simulink model "CARTESIAN_SPACE"  (R2021a)
settings: Solver=FixedStepAuto  StartTime=0.0  StopTime=10  FixedStep=0.01  RelTol=1e-3
model workspace: external: MATLAB File D:\OneDrive\STUDY\RIC LAB\PROJECT 6DOF\CODE\CODE 6DOF\10_SIMSCAPE\03\ROBOT_DataFile.m (data not in the file)
values from neighbouring files (symbols this model uses):
  circle = zeros(10/step+1,7)    [CIRCLE_01.m]
undefined symbols (not defined in the file or in its folder): smiData, X, Y, Z
libraries: sm_lib x36, nesl_utility x13
(part 2 of 3)

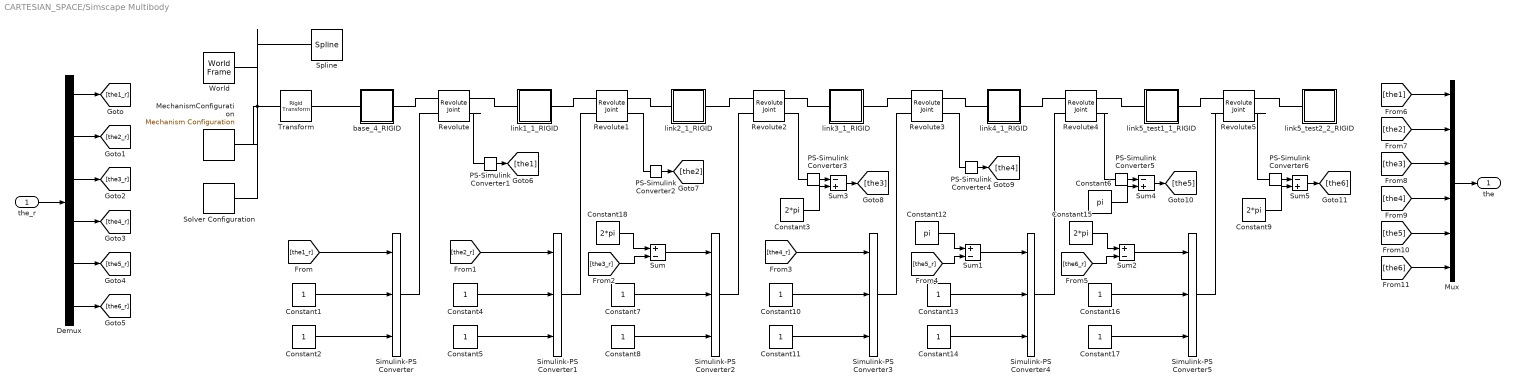
== system CARTESIAN_SPACE/Simscape Multibody ==
  the_r : Inport
  Constant{1..2,4..5,7..8,10..11,13..14,16..17} (12 alike) : Constant
  Constant12 : Constant  Value=pi
  Constant{3,9,15,18} (4 alike) : Constant  Value=2*pi
  Constant6 : Constant  Value=pi
  Demux : Demux  Outputs=6
  MechanismConfiguration : sm_lib/Utilities/Mechanism Configuration  UniformGravity=Constant  GravityVector=[0 -9.80665 0]  GravityVectorUnits=m/s^2  GravityUnits=m/s^2  LinearizationDelta=0.001  JointModeTransitionNonlinearIterations=2
  Mux : Mux  Inputs=6
  PS-Simulink Converter{1..6} (6 alike) : nesl_utility/PS-Simulink Converter  PhysicalDomain=network_engine_domain  SubClassName=ps_output  LeftPortType=input  RightPortType=output  PseudoPeriodic=off  Frequencies=[]  Unit=inherit  AffineConversion=off
      settings: SourceProductBaseCode=PW,SS
  Revolute : sm_lib/Joints/Revolute Joint  JointMode=Normal  SenseConstraintForce=off  SenseConstraintForceX=off  SenseConstraintForceY=off  SenseConstraintForceZ=off  SenseConstraintTorque=off  SenseConstraintTorqueX=off  SenseConstraintTorqueY=off  SenseConstraintTorqueZ=off  SenseTotalForce=off  SenseTotalForceX=off  SenseTotalForceY=off  SenseTotalForceZ=off  SenseTotalTorque=off  SenseTotalTorqueX=off  SenseTotalTorqueY=off  SenseTotalTorqueZ=off  CompositeWrenchDir=FollowerOnBase  CompositeWrenchFrame=BaseFrame  EquilibriumPosition=0  EquilibriumPositionUnits=deg  SpringStiffness=0  SpringStiffnessUnits=N*m/deg  DampingCoefficient=0  DampingCoefficientUnits=N*m/(deg/s)  TorqueActuationMode=ComputedTorque  MotionActuationMode=InputMotion  SensePosition=on  SenseVelocity=off  SenseAcceleration=off  SenseTorqueForce=off  SenseLowerLimitTorqueForce=off  SenseUpperLimitTorqueForce=off  LowerLimitSpecify=off  LowerLimitBound=-90  LowerLimitBoundUnits=deg  LowerLimitStiffness=1e4  LowerLimitStiffnessUnits=N*m/deg  LowerLimitDamping=10  LowerLimitDampingUnits=N*m/(deg/s)  LowerLimitTransitionRegionWidth=0.1  LowerLimitTransitionRegionWidthUnits=deg  UpperLimitSpecify=off  UpperLimitBound=90  UpperLimitBoundUnits=deg  UpperLimitStiffness=1e4  UpperLimitStiffnessUnits=N*m/deg  UpperLimitDamping=10  UpperLimitDampingUnits=N*m/(deg/s)  UpperLimitTransitionRegionWidth=0.1  UpperLimitTransitionRegionWidthUnits=deg  PositionTargetSpecify=on  PositionTargetPriority=Low  PositionTargetValue=smiData.RevoluteJoint(2).Rz.Pos  PositionTargetValueUnits=deg  VelocityTargetSpecify=off  VelocityTargetPriority=High  VelocityTargetValue=0  VelocityTargetValueUnits=deg/s
  Revolute1 : sm_lib/Joints/Revolute Joint  JointMode=Normal  SenseConstraintForce=off  SenseConstraintForceX=off  SenseConstraintForceY=off  SenseConstraintForceZ=off  SenseConstraintTorque=off  SenseConstraintTorqueX=off  SenseConstraintTorqueY=off  SenseConstraintTorqueZ=off  SenseTotalForce=off  SenseTotalForceX=off  SenseTotalForceY=off  SenseTotalForceZ=off  SenseTotalTorque=off  SenseTotalTorqueX=off  SenseTotalTorqueY=off  SenseTotalTorqueZ=off  CompositeWrenchDir=FollowerOnBase  CompositeWrenchFrame=BaseFrame  EquilibriumPosition=0  EquilibriumPositionUnits=deg  SpringStiffness=0  SpringStiffnessUnits=N*m/deg  DampingCoefficient=0  DampingCoefficientUnits=N*m/(deg/s)  TorqueActuationMode=ComputedTorque  MotionActuationMode=InputMotion  SensePosition=on  SenseVelocity=off  SenseAcceleration=off  SenseTorqueForce=off  SenseLowerLimitTorqueForce=off  SenseUpperLimitTorqueForce=off  LowerLimitSpecify=off  LowerLimitBound=-90  LowerLimitBoundUnits=deg  LowerLimitStiffness=1e4  LowerLimitStiffnessUnits=N*m/deg  LowerLimitDamping=10  LowerLimitDampingUnits=N*m/(deg/s)  LowerLimitTransitionRegionWidth=0.1  LowerLimitTransitionRegionWidthUnits=deg  UpperLimitSpecify=off  UpperLimitBound=90  UpperLimitBoundUnits=deg  UpperLimitStiffness=1e4  UpperLimitStiffnessUnits=N*m/deg  UpperLimitDamping=10  UpperLimitDampingUnits=N*m/(deg/s)  UpperLimitTransitionRegionWidth=0.1  UpperLimitTransitionRegionWidthUnits=deg  PositionTargetSpecify=on  PositionTargetPriority=Low  PositionTargetValue=smiData.RevoluteJoint(1).Rz.Pos  PositionTargetValueUnits=deg  VelocityTargetSpecify=off  VelocityTargetPriority=High  VelocityTargetValue=0  VelocityTargetValueUnits=deg/s
  Revolute2 : sm_lib/Joints/Revolute Joint  JointMode=Normal  SenseConstraintForce=off  SenseConstraintForceX=off  SenseConstraintForceY=off  SenseConstraintForceZ=off  SenseConstraintTorque=off  SenseConstraintTorqueX=off  SenseConstraintTorqueY=off  SenseConstraintTorqueZ=off  SenseTotalForce=off  SenseTotalForceX=off  SenseTotalForceY=off  SenseTotalForceZ=off  SenseTotalTorque=off  SenseTotalTorqueX=off  SenseTotalTorqueY=off  SenseTotalTorqueZ=off  CompositeWrenchDir=FollowerOnBase  CompositeWrenchFrame=BaseFrame  EquilibriumPosition=0  EquilibriumPositionUnits=deg  SpringStiffness=0  SpringStiffnessUnits=N*m/deg  DampingCoefficient=0  DampingCoefficientUnits=N*m/(deg/s)  TorqueActuationMode=ComputedTorque  MotionActuationMode=InputMotion  SensePosition=on  SenseVelocity=off  SenseAcceleration=off  SenseTorqueForce=off  SenseLowerLimitTorqueForce=off  SenseUpperLimitTorqueForce=off  LowerLimitSpecify=off  LowerLimitBound=-90  LowerLimitBoundUnits=deg  LowerLimitStiffness=1e4  LowerLimitStiffnessUnits=N*m/deg  LowerLimitDamping=10  LowerLimitDampingUnits=N*m/(deg/s)  LowerLimitTransitionRegionWidth=0.1  LowerLimitTransitionRegionWidthUnits=deg  UpperLimitSpecify=off  UpperLimitBound=90  UpperLimitBoundUnits=deg  UpperLimitStiffness=1e4  UpperLimitStiffnessUnits=N*m/deg  UpperLimitDamping=10  UpperLimitDampingUnits=N*m/(deg/s)  UpperLimitTransitionRegionWidth=0.1  UpperLimitTransitionRegionWidthUnits=deg  PositionTargetSpecify=on  PositionTargetPriority=Low  PositionTargetValue=smiData.RevoluteJoint(3).Rz.Pos  PositionTargetValueUnits=deg  VelocityTargetSpecify=off  VelocityTargetPriority=High  VelocityTargetValue=0  VelocityTargetValueUnits=deg/s
  Revolute3 : sm_lib/Joints/Revolute Joint  JointMode=Normal  SenseConstraintForce=off  SenseConstraintForceX=off  SenseConstraintForceY=off  SenseConstraintForceZ=off  SenseConstraintTorque=off  SenseConstraintTorqueX=off  SenseConstraintTorqueY=off  SenseConstraintTorqueZ=off  SenseTotalForce=off  SenseTotalForceX=off  SenseTotalForceY=off  SenseTotalForceZ=off  SenseTotalTorque=off  SenseTotalTorqueX=off  SenseTotalTorqueY=off  SenseTotalTorqueZ=off  CompositeWrenchDir=FollowerOnBase  CompositeWrenchFrame=BaseFrame  EquilibriumPosition=0  EquilibriumPositionUnits=deg  SpringStiffness=0  SpringStiffnessUnits=N*m/deg  DampingCoefficient=0  DampingCoefficientUnits=N*m/(deg/s)  TorqueActuationMode=ComputedTorque  MotionActuationMode=InputMotion  SensePosition=on  SenseVelocity=off  SenseAcceleration=off  SenseTorqueForce=off  SenseLowerLimitTorqueForce=off  SenseUpperLimitTorqueForce=off  LowerLimitSpecify=off  LowerLimitBound=-90  LowerLimitBoundUnits=deg  LowerLimitStiffness=1e4  LowerLimitStiffnessUnits=N*m/deg  LowerLimitDamping=10  LowerLimitDampingUnits=N*m/(deg/s)  LowerLimitTransitionRegionWidth=0.1  LowerLimitTransitionRegionWidthUnits=deg  UpperLimitSpecify=off  UpperLimitBound=90  UpperLimitBoundUnits=deg  UpperLimitStiffness=1e4  UpperLimitStiffnessUnits=N*m/deg  UpperLimitDamping=10  UpperLimitDampingUnits=N*m/(deg/s)  UpperLimitTransitionRegionWidth=0.1  UpperLimitTransitionRegionWidthUnits=deg  PositionTargetSpecify=on  PositionTargetPriority=Low  PositionTargetValue=smiData.RevoluteJoint(4).Rz.Pos  PositionTargetValueUnits=deg  VelocityTargetSpecify=off  VelocityTargetPriority=High  VelocityTargetValue=0  VelocityTargetValueUnits=deg/s
  Revolute4 : sm_lib/Joints/Revolute Joint  JointMode=Normal  SenseConstraintForce=off  SenseConstraintForceX=off  SenseConstraintForceY=off  SenseConstraintForceZ=off  SenseConstraintTorque=off  SenseConstraintTorqueX=off  SenseConstraintTorqueY=off  SenseConstraintTorqueZ=off  SenseTotalForce=off  SenseTotalForceX=off  SenseTotalForceY=off  SenseTotalForceZ=off  SenseTotalTorque=off  SenseTotalTorqueX=off  SenseTotalTorqueY=off  SenseTotalTorqueZ=off  CompositeWrenchDir=FollowerOnBase  CompositeWrenchFrame=BaseFrame  EquilibriumPosition=0  EquilibriumPositionUnits=deg  SpringStiffness=0  SpringStiffnessUnits=N*m/deg  DampingCoefficient=0  DampingCoefficientUnits=N*m/(deg/s)  TorqueActuationMode=ComputedTorque  MotionActuationMode=InputMotion  SensePosition=on  SenseVelocity=off  SenseAcceleration=off  SenseTorqueForce=off  SenseLowerLimitTorqueForce=off  SenseUpperLimitTorqueForce=off  LowerLimitSpecify=off  LowerLimitBound=-90  LowerLimitBoundUnits=deg  LowerLimitStiffness=1e4  LowerLimitStiffnessUnits=N*m/deg  LowerLimitDamping=10  LowerLimitDampingUnits=N*m/(deg/s)  LowerLimitTransitionRegionWidth=0.1  LowerLimitTransitionRegionWidthUnits=deg  UpperLimitSpecify=off  UpperLimitBound=90  UpperLimitBoundUnits=deg  UpperLimitStiffness=1e4  UpperLimitStiffnessUnits=N*m/deg  UpperLimitDamping=10  UpperLimitDampingUnits=N*m/(deg/s)  UpperLimitTransitionRegionWidth=0.1  UpperLimitTransitionRegionWidthUnits=deg  PositionTargetSpecify=on  PositionTargetPriority=Low  PositionTargetValue=smiData.RevoluteJoint(5).Rz.Pos  PositionTargetValueUnits=deg  VelocityTargetSpecify=off  VelocityTargetPriority=High  VelocityTargetValue=0  VelocityTargetValueUnits=deg/s
  Revolute5 : sm_lib/Joints/Revolute Joint  JointMode=Normal  SenseConstraintForce=off  SenseConstraintForceX=off  SenseConstraintForceY=off  SenseConstraintForceZ=off  SenseConstraintTorque=off  SenseConstraintTorqueX=off  SenseConstraintTorqueY=off  SenseConstraintTorqueZ=off  SenseTotalForce=off  SenseTotalForceX=off  SenseTotalForceY=off  SenseTotalForceZ=off  SenseTotalTorque=off  SenseTotalTorqueX=off  SenseTotalTorqueY=off  SenseTotalTorqueZ=off  CompositeWrenchDir=FollowerOnBase  CompositeWrenchFrame=BaseFrame  EquilibriumPosition=0  EquilibriumPositionUnits=deg  SpringStiffness=0  SpringStiffnessUnits=N*m/deg  DampingCoefficient=0  DampingCoefficientUnits=N*m/(deg/s)  TorqueActuationMode=ComputedTorque  MotionActuationMode=InputMotion  SensePosition=on  SenseVelocity=off  SenseAcceleration=off  SenseTorqueForce=off  SenseLowerLimitTorqueForce=off  SenseUpperLimitTorqueForce=off  LowerLimitSpecify=off  LowerLimitBound=-90  LowerLimitBoundUnits=deg  LowerLimitStiffness=1e4  LowerLimitStiffnessUnits=N*m/deg  LowerLimitDamping=10  LowerLimitDampingUnits=N*m/(deg/s)  LowerLimitTransitionRegionWidth=0.1  LowerLimitTransitionRegionWidthUnits=deg  UpperLimitSpecify=off  UpperLimitBound=90  UpperLimitBoundUnits=deg  UpperLimitStiffness=1e4  UpperLimitStiffnessUnits=N*m/deg  UpperLimitDamping=10  UpperLimitDampingUnits=N*m/(deg/s)  UpperLimitTransitionRegionWidth=0.1  UpperLimitTransitionRegionWidthUnits=deg  PositionTargetSpecify=on  PositionTargetPriority=Low  PositionTargetValue=smiData.RevoluteJoint(6).Rz.Pos  PositionTargetValueUnits=deg  VelocityTargetSpecify=off  VelocityTargetPriority=High  VelocityTargetValue=0  VelocityTargetValueUnits=deg/s
  Simulink-PS Converter{,1..5} (6 alike) : nesl_utility/Simulink-PS Converter  PhysicalDomain=network_engine_domain  SubClassName=ps_input  LeftPortType=input  RightPortType=output  PseudoPeriodic=off  Frequencies=[]  NoiseDistribution=none  NoiseParameters=[]  Unit=1  AffineConversion=off  FilteringAndDerivatives=provide  SimscapeFilterOrder=1  InputFilterTimeConstant=0.001  UdotUserProvided=2
      settings: SourceProductBaseCode=PW,SS
  Solver Configuration : nesl_utility/Solver Configuration  PhysicalDomain=network_engine_domain  SubClassName=solver  LeftPortType=input  RightPortType=generic  Tones=[]  Harmonics=[]  SimulateNoise=off  Profile=off  UseLocalSampling=off  EnableSwitchedLinearOptims=on  FrequencyDomain=off  UseCCode=off  RelTol=0.001  AbsTol=1e-06  MinStep=1e-09  ToWorkspace=off  RevertToSquareIcSolve=off  NumHomotopyIterations=100  PhasorMode=off  PhasorModeNumHarmonics=1  DoDC=off  ResidualTolerance=1e-09  UseLocalSolver=off  LocalSolverChoice=NE_BACKWARD_EULER_ADVANCER  LocalSolverSampleTime=0.001  DoFixedCost=off  MaxNonlinIter=3  MaxModeIter=2  ComputeImpulses=off  ImpulseIterations=2  LinearAlgebra=auto  EquationFormulation=NE_TIME_EF  DelaysMemoryBudget=1024  AutomaticFiltering=on  FilteringTimeConstant=0.001  PartitionStorageMethod=AS_NEEDED  PartitionMemoryBudget=1024  PartitionMethod=ROBUST
      settings: SourceProductBaseCode=PW,SS
  Spline : sm_lib/Curves and Surfaces/Spline  GraphicAmbientColor=[0.15 0.15 0.15 1.0]  GraphicDiffuseColor=[0.0 0.0 0.0]  DataPoints=|  DataPointsUnits=mm  GraphicEmissiveColor=[0.0 0.0 0.0 1.0]  EndConditionType=Natural  MarkerShape=Sphere  MarkerSize=10  GraphicType=FromGeometry  GraphicOpacity=1.0  GraphicShininess=75  GraphicSpecularColor=[0.5 0.5 0.5 1.0]  GraphicVisPropType=SimpleVisualProperties
      | [450.0000 -100.0000  650.0000
      |   450.0000  -99.9946  650.0000
      |   450.0000  -99.9785  650.0000
      |   450.0000  -99.9517  650.0000
      |   450.0000  -99.9143  650.0000
      |   450.0000  -99.8663  650.0000
      |   450.0000  -99.8079  650.0000
      |   450.0000  -99.7391  650.0000
      |   450.0000  -99.6599  650.0000
      |   450.0000  -99.5705  650.0000
      |   450.0000  -99.4708  650.0000
      |   450.0000  -99.3610  650.0000
      |   450.0000  -99.2411  650.0000
      |   450.0000  -99.1111  650.0000
      |   450.0000  -98.9712  650.0000
      |   450.0000  -98.8214  650.0000
      |   450.0000  -98.6618  650.0000
      |   450.0000  -98.4925  650.0000
      |   450.0000  -98.3134  650.0000
      |   450.0000  -98.1247  650.0000
      |   450.0000  -97.9264  650.0000
      |   450.0000  -97.7186  650.0000
      |   450.0000  -97.5014  650.0000
      |   450.0000  -97.2748  650.0000
      |   450.0000  -97.0389  650.0000
      |   450.0000  -96.7938  650.0000
      |   450.0000  -96.5394  650.0000
      |   450.0000  -96.2760  650.0000
      |   450.0000  -96.0035  650.0000
      |   450.0000  -95.7220  650.0000
      |   450.0000  -95.4316  650.0000
      |   450.0000  -95.1323  650.0000
      |   450.0000  -94.8243  650.0000
      |   450.0000  -94.5075  650.0000
      |   450.0000  -94.1821  650.0000
      |   450.0000  -93.8481  650.0000
      |   450.0000  -93.5055  650.0000
      |   450.0000  -93.1545  650.0000
      |   450.0000  -92.7950  650.0000
      |   450.0000  -92.4272  650.0000
      |   450.0000  -92.0512  650.0000
      |   450.0000  -91.6669  650.0000
      |   450.0000  -91.2746  650.0000
      |   450.0000  -90.8741  650.0000
      |   450.0000  -90.4656  650.0000
      |   450.0000  -90.0491  650.0000
      |   450.0000  -89.6248  650.0000
      |   450.0000  -89.1927  650.0000
      |   450.0000  -88.7528  650.0000
      |   450.0000  -88.3052  650.0000
      |   450.0000  -87.8500  650.0000
      |   450.0000  -87.3872  650.0000
      |   450.0000  -86.9170  650.0000
      |   450.0000  -86.4393  650.0000
      |   450.0000  -85.9542  650.0000
      |   450.0000  -85.4619  650.0000
      |   450.0000  -84.9623  650.0000
      |   450.0000  -84.4555  650.0000
      |   450.0000  -83.9416  650.0000
      |   450.0000  -83.4207  650.0000
      |   450.0000  -82.8928  650.0000
      |   450.0000  -82.3580  650.0000
      |   450.0000  -81.8163  650.0000
      |   450.0000  -81.2679  650.0000
      |   450.0000  -80.7128  650.0000
      |   450.0000  -80.1509  650.0000
      |   450.0000  -79.5826  650.0000
      |   450.0000  -79.0076  650.0000
      |   450.0000  -78.4263  650.0000
      |   450.0000  -77.8385  650.0000
      |   450.0000  -77.2444  650.0000
      |   450.0000  -76.6440  650.0000
      |   450.0000  -76.0375  650.0000
      |   450.0000  -75.4248  650.0000
      |   450.0000  -74.8060  650.0000
      |   450.0000  -74.1813  650.0000
      |   450.0000  -73.5505  650.0000
      |   450.0000  -72.9140  650.0000
      |   450.0000  -72.2716  650.0000
      |   450.0000  -71.6234  650.0000
      |   450.0000  -70.9696  650.0000
      |   450.0000  -70.3102  650.0000
      |   450.0000  -69.6452  650.0000
      |   450.0000  -68.9747  650.0000
      |   450.0000  -68.2988  650.0000
      |   450.0000  -67.6176  650.0000
      |   450.0000  -66.9310  650.0000
      |   450.0000  -66.2392  650.0000
      |   450.0000  -65.5423  650.0000
      |   450.0000  -64.8403  650.0000
      |   450.0000  -64.1332  650.0000
      |   450.0000  -63.4212  650.0000
      |   450.0000  -62.7042  650.0000
      |   450.0000  -61.9825  650.0000
      |   450.0000  -61.2559  650.0000
      |   450.0000  -60.5247  650.0000
      |   450.0000  -59.7887  650.0000
      |   450.0000  -59.0483  650.0000
      |   450.0000  -58.3033  650.0000
      |   450.0000  -57.5538  650.0000
      |   450.0000  -56.8000  650.0000
      |   450.0000  -56.0419  650.0000
      |   450.0000  -55.2794  650.0000
      |   450.0000  -54.5129  650.0000
      |   450.0000  -53.7421  650.0000
      |   450.0000  -52.9674  650.0000
      |   450.0000  -52.1886  650.0000
      |   450.0000  -51.4059  650.0000
      |   450.0000  -50.6193  650.0000
      |   450.0000  -49.8289  650.0000
      |   450.0000  -49.0348  650.0000
      |   450.0000  -48.2370  650.0000
      |   450.0000  -47.4356  650.0000
      |   450.0000  -46.6307  650.0000
      |   450.0000  -45.8223  650.0000
      |   450.0000  -45.0105  650.0000
      |   450.0000  -44.1953  650.0000
      |   450.0000  -43.3768  650.0000
      |   450.0000  -42.5551  650.0000
      |   450.0000  -41.7303  650.0000
      |   450.0000  -40.9024  650.0000
      |   450.0000  -40.0715  650.0000
      |   450.0000  -39.2376  650.0000
      |   450.0000  -38.4008  650.0000
      |   450.0000  -37.5611  650.0000
      |   450.0000  -36.7188  650.0000
      |   450.0000  -35.8737  650.0000
      |   450.0000  -35.0259  650.0000
      |   450.0000  -34.1756  650.0000
      |   450.0000  -33.3228  650.0000
      |   450.0000  -32.4676  650.0000
      |   450.0000  -31.6100  650.0000
      |   450.0000  -30.7501  650.0000
      |   450.0000  -29.8879  650.0000
      |   450.0000  -29.0235  650.0000
      |   450.0000  -28.1571  650.0000
      |   450.0000  -27.2885  650.0000
      |   450.0000  -26.4180  650.0000
      |   450.0000  -25.5456  650.0000
      |   450.0000  -24.6713  650.0000
      |   450.0000  -23.7952  650.0000
      |   450.0000  -22.9174  650.0000
      |   450.0000  -22.0379  650.0000
      |   450.0000  -21.1568  650.0000
      |   450.0000  -20.2742  650.0000
      |   450.0000  -19.3902  650.0000
      |   450.0000  -18.5047  650.0000
      |   450.0000  -17.6178  650.0000
      |   450.0000  -16.7298  650.0000
      |   450.0000  -15.8404  650.0000
      |   450.0000  -14.9500  650.0000
      |   450.0000  -14.0585  650.0000
      |   450.0000  -13.1659  650.0000
      |   450.0000  -12.2724  650.0000
      |   450.0000  -11.3781  650.0000
      |   450.0000  -10.4829  650.0000
      |   450.0000   -9.5869  650.0000
      |   450.0000   -8.6902  650.0000
      |   450.0000   -7.7930  650.0000
      |   450.0000   -6.8951  650.0000
      |   450.0000   -5.9968  650.0000
      |   450.0000   -5.0980  650.0000
      |   450.0000   -4.1989  650.0000
      |   450.0000   -3.2995  650.0000
      |   450.0000   -2.3998  650.0000
      |   450.0000   -1.5000  650.0000
      |   450.0000   -0.6000  650.0000
      |   450.0000    0.3000  650.0000
      |   450.0000    1.2000  650.0000
      |   450.0000    2.0999  650.0000
      |   450.0000    2.9996  650.0000
      |   450.0000    3.8991  650.0000
      |   450.0000    4.7984  650.0000
      |   450.0000    5.6973  650.0000
      |   450.0000    6.5957  650.0000
      |   450.0000    7.4937  650.0000
      |   450.0000    8.3912  650.0000
      |   450.0000    9.2881  650.0000
      |   450.0000   10.1843  650.0000
      |   450.0000   11.0797  650.0000
      |   450.0000   11.9744  650.0000
      |   450.0000   12.8682  650.0000
      |   450.0000   13.7611  650.0000
      |   450.0000   14.6529  650.0000
      |   450.0000   15.5438  650.0000
      |   450.0000   16.4334  650.0000
      |   450.0000   17.3220  650.0000
      |   450.0000   18.2092  650.0000
      |   450.0000   19.0951  650.0000
      |   450.0000   19.9797  650.0000
      |   450.0000   20.8628  650.0000
      |   450.0000   21.7444  650.0000
      |   450.0000   22.6244  650.0000
      |   450.0000   23.5028  650.0000
      |   450.0000   24.3795  650.0000
      |   450.0000   25.2543  650.0000
      |   450.0000   26.1274  650.0000
      |   450.0000   26.9986  650.0000
      |   450.0000   27.8678  650.0000
      |   450.0000   28.7349  650.0000
      |   450.0000   29.6000  650.0000
      |   450.0000   30.4629  650.0000
      |   450.0000   31.3236  650.0000
      |   450.0000   32.1820  650.0000
      |   450.0000   33.0380  650.0000
      |   450.0000   33.8916  650.0000
      |   450.0000   34.7428  650.0000
      |   450.0000   35.5914  650.0000
      |   450.0000   36.4374  650.0000
      |   450.0000   37.2806  650.0000
      |   450.0000   38.1212  650.0000
      |   450.0000   38.9589  650.0000
      |   450.0000   39.7938  650.0000
      |   450.0000   40.6258  650.0000
      |   450.0000   41.4547  650.0000
      |   450.0000   42.2805  650.0000
      |   450.0000   43.1033  650.0000
      |   450.0000   43.9228  650.0000
      |   450.0000   44.7391  650.0000
      |   450.0000   45.5520  650.0000
      |   450.0000   46.3616  650.0000
      |   450.0000   47.1677  650.0000
      |   450.0000   47.9703  650.0000
      |   450.0000   48.7693  650.0000
      |   450.0000   49.5646  650.0000
      |   450.0000   50.3562  650.0000
      |   450.0000   51.1441  650.0000
      |   450.0000   51.9281  650.0000
      |   450.0000   52.7082  650.0000
      |   450.0000   53.4843  650.0000
      |   450.0000   54.2564  650.0000
      |   450.0000   55.0244  650.0000
      |   450.0000   55.7882  650.0000
      |   450.0000   56.5478  650.0000
      |   450.0000   57.3030  650.0000
      |   450.0000   58.0539  650.0000
      |   450.0000   58.8004  650.0000
      |   450.0000   59.5424  650.0000
      |   450.0000   60.2799  650.0000
      |   450.0000   61.0127  650.0000
      |   450.0000   61.7408  650.0000
      |   450.0000   62.4642  650.0000
      |   450.0000   63.1827  650.0000
      |   450.0000   63.8964  650.0000
      |   450.0000   64.6051  650.0000
      |   450.0000   65.3088  650.0000
      |   450.0000   66.0075  650.0000
      |   450.0000   66.7010  650.0000
      |   450.0000   67.3893  650.0000
      |   450.0000   68.0723  650.0000
      |   450.0000   68.7500  650.0000
      |   450.0000   69.4223  650.0000
      |   450.0000   70.0891  650.0000
      |   450.0000   70.7504  650.0000
      |   450.0000   71.4061  650.0000
      |   450.0000   72.0561  650.0000
      |   450.0000   72.7005  650.0000
      |   450.0000   73.3390  650.0000
      |   450.0000   73.9717  650.0000
      |   450.0000   74.5984  650.0000
      |   450.0000   75.2192  650.0000
      |   450.0000   75.8339  650.0000
      |   450.0000   76.4425  650.0000
      |   450.0000   77.0450  650.0000
      |   450.0000   77.6412  650.0000
      |   450.0000   78.2310  650.0000
      |   450.0000   78.8146  650.0000
      |   450.0000   79.3916  650.0000
      |   450.0000   79.9622  650.0000
      |   450.0000   80.5262  650.0000
      |   450.0000   81.0836  650.0000
      |   450.0000   81.6343  650.0000
      |   450.0000   82.1782  650.0000
      |   450.0000   82.7153  650.0000
      |   450.0000   83.2455  650.0000
      |   450.0000   83.7687  650.0000
      |   450.0000   84.2850  650.0000
      |   450.0000   84.7941  650.0000
      |   450.0000   85.2961  650.0000
      |   450.0000   85.7909  650.0000
      |   450.0000   86.2784  650.0000
      |   450.0000   86.7586  650.0000
      |   450.0000   87.2313  650.0000
      |   450.0000   87.6966  650.0000
      |   450.0000   88.1543  650.0000
      |   450.0000   88.6044  650.0000
      |   450.0000   89.0469  650.0000
      |   450.0000   89.4816  650.0000
      |   450.0000   89.9086  650.0000
      |   450.0000   90.3277  650.0000
      |   450.0000   90.7388  650.0000
      |   450.0000   91.1420  650.0000
      |   450.0000   91.5370  650.0000
      |   450.0000   91.9240  650.0000
      |   450.0000   92.3028  650.0000
      |   450.0000   92.6733  650.0000
      |   450.0000   93.0356  650.0000
      |   450.0000   93.3894  650.0000
      |   450.0000   93.7348  650.0000
      |   450.0000   94.0717  650.0000
      |   450.0000   94.4000  650.0000
      |   450.0000   94.7197  650.0000
      |   450.0000   95.0306  650.0000
      |   450.0000   95.3328  650.0000
      |   450.0000   95.6262  650.0000
      |   450.0000   95.9106  650.0000
      |   450.0000   96.1861  650.0000
      |   450.0000   96.4526  650.0000
      |   450.0000   96.7100  650.0000
      |   450.0000   96.9582  650.0000
      |   450.0000   97.1972  650.0000
      |   450.0000   97.4269  650.0000
      |   450.0000   97.6473  650.0000
      |   450.0000   97.8582  650.0000
      |   450.0000   98.0596  650.0000
      |   450.0000   98.2515  650.0000
      |   450.0000   98.4338  650.0000
      |   450.0000   98.6065  650.0000
      |   450.0000   98.7693  650.0000
      |   450.0000   98.9224  650.0000
      |   450.0000   99.0656  650.0000
      |   450.0000   99.1989  650.0000
      |   450.0000   99.3221  650.0000
      |   450.0000   99.4353  650.0000
      |   450.0000   99.5384  650.0000
      |   450.0000   99.6312  650.0000
      |   450.0000   99.7139  650.0000
      |   450.0000   99.7861  650.0000
      |   450.0000   99.8480  650.0000
      |   450.0000   99.8995  650.0000
      |   450.0000   99.9404  650.0000
      |   450.0000   99.9707  650.0000
      |   450.0000   99.9904  650.0000
      |   450.0000   99.9994  650.0000
      |   450.0000   99.9988  649.9982
      |   450.0000   99.9925  649.9888
      |   450.0000   99.9809  649.9714
      |   450.0000   99.9640  649.9459
      |   450.0000   99.9417  649.9126
      |   450.0000   99.9143  649.8714
      |   450.0000   99.8816  649.8224
      |   450.0000   99.8437  649.7656
      |   450.0000   99.8007  649.7011
      |   450.0000   99.7526  649.6289
      |   450.0000   99.6994  649.5490
      |   450.0000   99.6411  649.4616
      |   450.0000   99.5778  649.3667
      |   450.0000   99.5095  649.2642
      |   450.0000   99.4362  649.1544
      |   450.0000   99.3581  649.0371
      |   450.0000   99.2750  648.9125
      |   450.0000   99.1871  648.7806
      |   450.0000   99.0943  648.6415
      |   450.0000   98.9968  648.4952
      |   450.0000   98.8945  648.3417
      |   450.0000   98.7874  648.1811
      |   450.0000   98.6757  648.0135
      |   450.0000   98.5593  647.8389
      |   450.0000   98.4382  647.6574
      |   450.0000   98.3126  647.4689
      |   450.0000   98.1824  647.2736
      |   450.0000   98.0477  647.0715
      |   450.0000   97.9084  646.8626
      |   450.0000   97.7647  646.6470
      |   450.0000   97.6165  646.4248
      |   450.0000   97.4640  646.1960
      |   450.0000   97.3070  645.9606
      |   450.0000   97.1458  645.7186
      |   450.0000   96.9802  645.4703
      |   450.0000   96.8103  645.2155
      |   450.0000   96.6362  644.9543
      |   450.0000   96.4579  644.6868
      |   450.0000   96.2754  644.4131
      |   450.0000   96.0887  644.1331
      |   450.0000   95.8980  643.8470
      |   450.0000   95.7031  643.5547
      |   450.0000   95.5042  643.2563
      |   450.0000   95.3013  642.9520
      |   450.0000   95.0944  642.6416
      |   450.0000   94.8836  642.3254
      |   450.0000   94.6688  642.0032
      |   450.0000   94.4501  641.6752
      |   450.0000   94.2276  641.3414
      |   450.0000   94.0013  641.0019
      |   450.0000   93.7712  640.6567
      |   450.0000   93.5373  640.3059
      |   450.0000   93.2997  639.9495
      |   450.0000   93.0584  639.5875
      |   450.0000   92.8134  639.2201
      |   450.0000   92.5648  638.8472
      |   450.0000   92.3126  638.4689
      |   450.0000   92.0568  638.0853
      |   450.0000   91.7976  637.6963
      |   450.0000   91.5348  637.3022
      |   450.0000   91.2685  636.9028
      |   450.0000   90.9988  636.4982
      |   450.0000   90.7257  636.0886
      |   450.0000   90.4493  635.6739
      |   450.0000   90.1695  635.2542
      |   450.0000   89.8864  634.8296
      |   450.0000   89.6000  634.4000
      |   450.0000   89.3104  633.9656
      |   450.0000   89.0176  633.5263
      |   450.0000   88.7216  633.0823
      |   450.0000   88.4224  632.6336
      |   450.0000   88.1202  632.1803
      |   450.0000   87.8148  631.7223
      |   450.0000   87.5065  631.2597
      |   450.0000   87.1951  630.7926
      |   450.0000   86.8807  630.3211
      |   450.0000   86.5634  629.8451
      |   450.0000   86.2432  629.3648
      |   450.0000   85.9201  628.8801
      |   450.0000   85.5941  628.3911
      |   450.0000   85.2653  627.8979
      |   450.0000   84.9337  627.4006
      |   450.0000   84.5994  626.8991
      |   450.0000   84.2624  626.3935
      |   450.0000   83.9226  625.8839
      |   450.0000   83.5802  625.3703
      |   450.0000   83.2352  624.8528
      |   450.0000   82.8876  624.3314
      |   450.0000   82.5374  623.8061
      |   450.0000   82.1847  623.2771
      |   450.0000   81.8295  622.7443
      |   450.0000   81.4719  622.2078
      |   450.0000   81.1118  621.6677
      |   450.0000   80.7493  621.1240
      |   450.0000   80.3845  620.5767
      |   450.0000   80.0173  620.0259
      |   450.0000   79.6478  619.4717
      |   450.0000   79.2761  618.9141
      |   450.0000   78.9021  618.3531
      |   450.0000   78.5259  617.7888
      |   450.0000   78.1475  617.2213
      |   450.0000   77.7670  616.6505
      |   450.0000   77.3844  616.0766
      |   450.0000   76.9997  615.4996
      |   450.0000   76.6130  614.9195
      |   450.0000   76.2243  614.3365
      |   450.0000   75.8336  613.7504
      |   450.0000   75.4410  613.1614
      |   450.0000   75.0464  612.5696
      |   450.0000   74.6500  611.9749
      |   450.0000   74.2517  611.3775
      |   450.0000   73.8516  610.7774
      |   450.0000   73.4497  610.1745
      |   450.0000   73.0461  609.5691
      |   450.0000   72.6407  608.9611
      |   450.0000   72.2337  608.3505
      |   450.0000   71.8250  607.7375
      |   450.0000   71.4147  607.1220
      |   450.0000   71.0028  606.5042
      |   450.0000   70.5894  605.8840
      |   450.0000   70.1744  605.2616
      |   450.0000   69.7579  604.6369
      |   450.0000   69.3400  604.0100
      |   450.0000   68.9207  603.3810
      |   450.0000   68.4999  602.7499
      |   450.0000   68.0778  602.1167
      |   450.0000   67.6544  601.4816
      |   450.0000   67.2297  600.8445
      |   450.0000   66.8037  600.2055
      |   450.0000   66.3765  599.5647
      |   450.0000   65.9481  598.9221
      |   450.0000   65.5185  598.2777
      |   450.0000   65.0878  597.6316
      |   450.0000   64.6559  596.9839
      |   450.0000   64.2231  596.3346
      |   450.0000   63.7891  595.6837
      |   450.0000   63.3542  595.0313
      |   450.0000   62.9183  594.3774
      |   450.0000   62.4815  593.7222
      |   450.0000   62.0437  593.0656
      |   450.0000   61.6051  592.4076
      |   450.0000   61.1656  591.7484
      |   450.0000   60.7254  591.0880
      |   450.0000   60.2843  590.4264
      |   450.0000   59.8425  589.7638
      |   450.0000   59.4000  589.1000
      |   450.0000   58.9568  588.4352
      |   450.0000   58.5130  587.7694
      |   450.0000   58.0685  587.1028
      |   450.0000   57.6235  586.4352
      |   450.0000   57.1779  585.7668
      |   450.0000   56.7318  585.0977
      |   450.0000   56.2852  584.4278
      |   450.0000   55.8381  583.7572
      |   450.0000   55.3907  583.0860
      |   450.0000   54.9428  582.4142
      |   450.0000   54.4946  581.7419
      |   450.0000   54.0461  581.0691
      |   450.0000   53.5972  580.3959
      |   450.0000   53.1481  579.7222
      |   450.0000   52.6988  579.0483
      |   450.0000   52.2493  578.3740
      |   450.0000   51.7997  577.6995
      |   450.0000   51.3499  577.0248
      |   450.0000   50.9000  576.3499
      |   450.0000   50.4500  575.6750
      |   450.0000   50.0000  575.0000
      |   450.0000   49.5500  574.3250
      |   450.0000   49.1000  573.6501
      |   450.0000   48.6501  572.9752
      |   450.0000   48.2003  572.3005
      |   450.0000   47.7507  571.6260
      |   450.0000   47.3012  570.9517
      |   450.0000   46.8519  570.2778
      |   450.0000   46.4028  569.6041
      |   450.0000   45.9539  568.9309
      |   450.0000   45.5054  568.2581
      |   450.0000   45.0572  567.5858
      |   450.0000   44.6093  566.9140
      |   450.0000   44.1619  566.2428
      |   450.0000   43.7148  565.5722
      |   450.0000   43.2682  564.9023
      |   450.0000   42.8221  564.2332
      |   450.0000   42.3765  563.5648
      |   450.0000   41.9315  562.8972
      |   450.0000   41.4870  562.2306
      |   450.0000   41.0432  561.5648
      |   450.0000   40.6000  560.9000
      |   450.0000   40.1575  560.2362
      |   450.0000   39.7157  559.5736
      |   450.0000   39.2746  558.9120
      |   450.0000   38.8344  558.2516
      |   450.0000   38.3949  557.5924
      |   450.0000   37.9563  556.9344
      |   450.0000   37.5185  556.2778
      |   450.0000   37.0817  555.6226
      |   450.0000   36.6458  554.9687
      |   450.0000   36.2109  554.3163
      |   450.0000   35.7769  553.6654
      |   450.0000   35.3441  553.0161
      |   450.0000   34.9122  552.3684
      |   450.0000   34.4815  551.7223
      |   450.0000   34.0519  551.0779
      |   450.0000   33.6235  550.4353
      |   450.0000   33.1963  549.7945
      |   450.0000   32.7703  549.1555
      |   450.0000   32.3456  548.5184
      |   450.0000   31.9222  547.8833
      |   450.0000   31.5001  547.2501
      |   450.0000   31.0793  546.6190
      |   450.0000   30.6600  545.9900
      |   450.0000   30.2421  545.3631
      |   450.0000   29.8256  544.7384
      |   450.0000   29.4106  544.1160
      |   450.0000   28.9972  543.4958
      |   450.0000   28.5853  542.8780
      |   450.0000   28.1750  542.2625
      |   450.0000   27.7663  541.6495
      |   450.0000   27.3593  541.0389
      |   450.0000   26.9539  540.4309
      |   450.0000   26.5503  539.8255
      |   450.0000   26.1484  539.2226
      |   450.0000   25.7483  538.6225
      |   450.0000   25.3500  538.0251
      |   450.0000   24.9536  537.4304
      |   450.0000   24.5590  536.8386
      |   450.0000   24.1664  536.2496
      |   450.0000   23.7757  535.6635
      |   450.0000   23.3870  535.0805
      |   450.0000   23.0003  534.5004
      |   450.0000   22.6156  533.9234
      |   450.0000   22.2330  533.3495
      |   450.0000   21.8525  532.7787
      |   450.0000   21.4741  532.2112
      |   450.0000   21.0979  531.6469
      |   450.0000   20.7239  531.0859
      |   450.0000   20.3522  530.5283
      |   450.0000   19.9827  529.9741
      |   450.0000   19.6155  529.4233
      |   450.0000   19.2507  528.8760
      |   450.0000   18.8882  528.3323
      |   450.0000   18.5281  527.7922
      |   450.0000   18.1705  527.2557
      |   450.0000   17.8153  526.7229
      |   450.0000   17.4626  526.1939
      |   450.0000   17.1124  525.6686
      |   450.0000   16.7648  525.1472
      |   450.0000   16.4198  524.6297
      |   450.0000   16.0774  524.1161
      |   450.0000   15.7376  523.6065
      |   450.0000   15.4006  523.1009
      |   450.0000   15.0663  522.5994
      |   450.0000   14.7347  522.1021
      |   450.0000   14.4059  521.6089
      |   450.0000   14.0799  521.1199
      |   450.0000   13.7568  520.6352
      |   450.0000   13.4366  520.1549
      |   450.0000   13.1193  519.6789
      |   450.0000   12.8049  519.2074
      |   450.0000   12.4935  518.7403
      |   450.0000   12.1852  518.2777
      |   450.0000   11.8798  517.8197
      |   450.0000   11.5776  517.3664
      |   450.0000   11.2784  516.9177
      |   450.0000   10.9824  516.4737
      |   450.0000   10.6896  516.0344
      |   450.0000   10.4000  515.6000
      |   450.0000   10.1136  515.1704
      |   450.0000    9.8305  514.7458
      |   450.0000    9.5507  514.3261
      |   450.0000    9.2743  513.9114
      |   450.0000    9.0012  513.5018
      |   450.0000    8.7315  513.0972
      |   450.0000    8.4652  512.6978
      |   450.0000    8.2024  512.3037
      |   450.0000    7.9432  511.9147
      |   450.0000    7.6874  511.5311
      |   450.0000    7.4352  511.1528
      |   450.0000    7.1866  510.7799
      |   450.0000    6.9416  510.4125
      |   450.0000    6.7003  510.0505
      |   450.0000    6.4627  509.6941
      |   450.0000    6.2288  509.3433
      |   450.0000    5.9987  508.9981
      |   450.0000    5.7724  508.6586
      |   450.0000    5.5499  508.3248
      |   450.0000    5.3312  507.9968
      |   450.0000    5.1164  507.6746
      |   450.0000    4.9056  507.3584
      |   450.0000    4.6987  507.0480
      |   450.0000    4.4958  506.7437
      |   450.0000    4.2969  506.4453
      |   450.0000    4.1020  506.1530
      |   450.0000    3.9113  505.8669
      |   450.0000    3.7246  505.5869
      |   450.0000    3.5421  505.3132
      |   450.0000    3.3638  505.0457
      |   450.0000    3.1897  504.7845
      |   450.0000    3.0198  504.5297
      |   450.0000    2.8542  504.2814
      |   450.0000    2.6930  504.0394
      |   450.0000    2.5360  503.8040
      |   450.0000    2.3835  503.5752
      |   450.0000    2.2353  503.3530
      |   450.0000    2.0916  503.1374
      |   450.0000    1.9523  502.9285
      |   450.0000    1.8176  502.7264
      |   450.0000    1.6874  502.5311
      |   450.0000    1.5618  502.3426
      |   450.0000    1.4407  502.1611
      |   450.0000    1.3243  501.9865
      |   450.0000    1.2126  501.8189
      |   450.0000    1.1055  501.6583
      |   450.0000    1.0032  501.5048
      |   450.0000    0.9057  501.3585
      |   450.0000    0.8129  501.2194
      |   450.0000    0.7250  501.0875
      |   450.0000    0.6419  500.9629
      |   450.0000    0.5638  500.8456
      |   450.0000    0.4905  500.7358
      |   450.0000    0.4222  500.6333
      |   450.0000    0.3589  500.5384
      |   450.0000    0.3006  500.4510
      |   450.0000    0.2474  500.3711
      |   450.0000    0.1993  500.2989
      |   450.0000    0.1563  500.2344
      |   450.0000    0.1184  500.1776
      |   450.0000    0.0857  500.1286
      |   450.0000    0.0583  500.0874
      |   450.0000    0.0360  500.0541
      |   450.0000    0.0191  500.0286
      |   450.0000    0.0075  500.0112
      |   450.0000    0.0012  500.0018
      |   450.0000   -0.0003  500.0004
      |   450.0000   -0.0048  500.0072
      |   450.0000   -0.0146  500.0219
      |   450.0000   -0.0298  500.0447
      |   450.0000   -0.0503  500.0754
      |   450.0000   -0.0760  500.1140
      |   450.0000   -0.1069  500.1604
      |   450.0000   -0.1431  500.2146
      |   450.0000   -0.1844  500.2766
      |   450.0000   -0.2308  500.3462
      |   450.0000   -0.2823  500.4235
      |   450.0000   -0.3389  500.5084
      |   450.0000   -0.4006  500.6009
      |   450.0000   -0.4672  500.7008
      |   450.0000   -0.5388  500.8082
      |   450.0000   -0.6153  500.9230
      |   450.0000   -0.6968  501.0452
      |   450.0000   -0.7831  501.1746
      |   450.0000   -0.8742  501.3113
      |   450.0000   -0.9702  501.4553
      |   450.0000   -1.0709  501.6064
      |   450.0000   -1.1764  501.7646
      |   450.0000   -1.2865  501.9298
      |   450.0000   -1.4014  502.1021
      |   450.0000   -1.5209  502.2813
      |   450.0000   -1.6450  502.4675
      |   450.0000   -1.7737  502.6605
      |   450.0000   -1.9069  502.8604
      |   450.0000   -2.0447  503.0670
      |   450.0000   -2.1869  503.2804
      |   450.0000   -2.3336  503.5004
      |   450.0000   -2.4847  503.7270
      |   450.0000   -2.6402  503.9602
      |   450.0000   -2.8000  504.2000
      |   450.0000   -2.9642  504.4462
      |   450.0000   -3.1326  504.6989
      |   450.0000   -3.3053  504.9579
      |   450.0000   -3.4822  505.2233
      |   450.0000   -3.6633  505.4950
      |   450.0000   -3.8486  505.7729
      |   450.0000   -4.0380  506.0570
      |   450.0000   -4.2315  506.3472
      |   450.0000   -4.4290  506.6435
      |   450.0000   -4.6306  506.9459
      |   450.0000   -4.8362  507.2543
      |   450.0000   -5.0457  507.5686
      |   450.0000   -5.2592  507.8888
      |   450.0000   -5.4765  508.2148
      |   450.0000   -5.6978  508.5467
      |   450.0000   -5.9228  508.8843
      |   450.0000   -6.1517  509.2276
      |   450.0000   -6.3843  509.5765
      |   450.0000   -6.6207  509.9311
      |   450.0000   -6.8608  510.2912
      |   450.0000   -7.1046  510.6568
      |   450.0000   -7.3519  511.0279
      |   450.0000   -7.6029  511.4044
      |   450.0000   -7.8575  511.7863
      |   450.0000   -8.1156  512.1734
      |   450.0000   -8.3772  512.5659
      |   450.0000   -8.6424  512.9635
      |   450.0000   -8.9109  513.3663
      |   450.0000   -9.1829  513.7743
      |   450.0000   -9.4582  514.1873
      |   450.0000   -9.7369  514.6053
      |   450.0000  -10.0189  515.0283
      |   450.0000  -10.3042  515.4563
      |   450.0000  -10.5927  515.8891
      |   450.0000  -10.8845  516.3267
      |   450.0000  -11.1794  516.7691
      |   450.0000  -11.4775  517.2163
      |   450.0000  -11.7787  517.6681
      |   450.0000  -12.0830  518.1246
      |   450.0000  -12.3904  518.5856
      |   450.0000  -12.7008  519.0512
      |   450.0000  -13.0142  519.5212
      |   450.0000  -13.3305  519.9958
      |   450.0000  -13.6498  520.4746
      |   450.0000  -13.9719  520.9579
      |   450.0000  -14.2969  521.4454
      |   450.0000  -14.6248  521.9372
      |   450.0000  -14.9554  522.4332
      |   450.0000  -15.2889  522.9333
      |   450.0000  -15.6250  523.4375
      |   450.0000  -15.9638  523.9458
      |   450.0000  -16.3054  524.4580
      |   450.0000  -16.6495  524.9743
      |   450.0000  -16.9963  525.4944
      |   450.0000  -17.3456  526.0184
      |   450.0000  -17.6974  526.5462
      |   450.0000  -18.0518  527.0777
      |   450.0000  -18.4086  527.6130
      |   450.0000  -18.7679  528.1519
      |   450.0000  -19.1296  528.6944
      |   450.0000  -19.4937  529.2405
      |   450.0000  -19.8601  529.7901
      |   450.0000  -20.2288  530.3432
      |   450.0000  -20.5998  530.8997
      |   450.0000  -20.9730  531.4595
      |   450.0000  -21.3485  532.0227
      |   450.0000  -21.7261  532.5892
      |   450.0000  -22.1059  533.1589
      |   450.0000  -22.4878  533.7317
      |   450.0000  -22.8718  534.3077
      |   450.0000  -23.2578  534.8868
      |   450.0000  -23.6459  535.4689
      |   450.0000  -24.0359  536.0539
      |   450.0000  -24.4280  536.6419
      |   450.0000  -24.8219  537.2328
      |   450.0000  -25.2177  537.8265
      |   450.0000  -25.6154  538.4230
      |   450.0000  -26.0149  539.0223
      |   450.0000  -26.4161  539.6242
      |   450.0000  -26.8192  540.2288
      |   450.0000  -27.2240  540.8360
      |   450.0000  -27.6305  541.4457
      |   450.0000  -28.0386  542.0579
      |   450.0000  -28.4484  542.6725
      |   450.0000  -28.8597  543.2896
      |   450.0000  -29.2727  543.9090
      |   450.0000  -29.6871  544.5307
      |   450.0000  -30.1031  545.1546
      |   450.0000  -30.5205  545.7808
      |   450.0000  -30.9394  546.4091
      |   450.0000  -31.3597  547.0395
      |   450.0000  -31.7813  547.6720
      |   450.0000  -32.2043  548.3065
      |   450.0000  -32.6286  548.9429
      |   450.0000  -33.0542  549.5813
      |   450.0000  -33.4810  550.2215
      |   450.0000  -33.9090  550.8635
      |   450.0000  -34.3382  551.5073
      |   450.0000  -34.7685  552.1528
      |   450.0000  -35.2000  552.8000
      |   450.0000  -35.6325  553.4488
      |   450.0000  -36.0661  554.0992
      |   450.0000  -36.5007  554.7511
      |   450.0000  -36.9363  555.4044
      |   450.0000  -37.3728  556.0592
      |   450.0000  -37.8103  556.7154
      |   450.0000  -38.2486  557.3729
      |   450.0000  -38.6878  558.0317
      |   450.0000  -39.1278  558.6917
      |   450.0000  -39.5686  559.3529
      |   450.0000  -40.0102  560.0152
      |   450.0000  -40.4524  560.6786
      |   450.0000  -40.8954  561.3431
      |   450.0000  -41.3390  562.0085
      |   450.0000  -41.7833  562.6749
      |   450.0000  -42.2281  563.3422
      |   450.0000  -42.6735  564.0103
      |   450.0000  -43.1195  564.6792
      |   450.0000  -43.5659  565.3489
      |   450.0000  -44.0128  566.0192
      |   450.0000  -44.4601  566.6902
      |   450.0000  -44.9079  567.3618
      |   450.0000  -45.3560  568.0339
      |   450.0000  -45.8044  568.7066
      |   450.0000  -46.2531  569.3797
      |   450.0000  -46.7021  570.0532
      |   450.0000  -47.1514  570.7271
      |   450.0000  -47.6008  571.4012
      |   450.0000  -48.0504  572.0757
      |   450.0000  -48.5002  572.7503
      |   450.0000  -48.9501  573.4251
      |   450.0000  -49.4000  574.1000
      |   450.0000  -49.8500  574.7750
      |   450.0000  -50.3000  575.4500
      |   450.0000  -50.7500  576.1250
      |   450.0000  -51.1999  576.7998
      |   450.0000  -51.6497  577.4746
      |   450.0000  -52.0995  578.1492
      |   450.0000  -52.5490  578.8235
      |   450.0000  -52.9984  579.4976
      |   450.0000  -53.4476  580.1713
      |   450.0000  -53.8965  580.8447
      |   450.0000  -54.3451  581.5177
      |   450.0000  -54.7934  582.1902
      |   450.0000  -55.2414  582.8621
      |   450.0000  -55.6890  583.5335
      |   450.0000  -56.1362  584.2043
      |   450.0000  -56.5830  584.8744
      |   450.0000  -57.0292  585.5439
      |   450.0000  -57.4750  586.2125
      |   450.0000  -57.9202  586.8803
      |   450.0000  -58.3649  587.5473
      |   450.0000  -58.8089  588.2134
      |   450.0000  -59.2523  588.8785
      |   450.0000  -59.6951  589.5426
      |   450.0000  -60.1371  590.2057
      |   450.0000  -60.5784  590.8676
      |   450.0000  -61.0190  591.5284
      |   450.0000  -61.4587  592.1880
      |   450.0000  -61.8976  592.8464
      |   450.0000  -62.3356  593.5035
      |   450.0000  -62.7728  594.1592
      |   450.0000  -63.2090  594.8135
      |   450.0000  -63.6443  595.4664
      |   450.0000  -64.0785  596.1178
      |   450.0000  -64.5118  596.7676
      |   450.0000  -64.9439  597.4159
      |   450.0000  -65.3750  598.0625
      |   450.0000  -65.8050  598.7075
      |   450.0000  -66.2338  599.3507
      |   450.0000  -66.6614  599.9921
      |   450.0000  -67.0878  600.6317
      |   450.0000  -67.5130  601.2695
      |   450.0000  -67.9368  601.9052
      |   450.0000  -68.3594  602.5391
      |   450.0000  -68.7806  603.1709
      |   450.0000  -69.2004  603.8006
      |   450.0000  -69.6188  604.4282
      |   450.0000  -70.0357  605.0536
      |   450.0000  -70.4512  605.6768
      |   450.0000  -70.8652  606.2977
      |   450.0000  -71.2776  606.9164
      |   450.0000  -71.6884  607.5326
      |   450.0000  -72.0976  608.1465
      |   450.0000  -72.5052  608.7578
      |   450.0000  -72.9111  609.3667
      |   450.0000  -73.3153  609.9730
      |   450.0000  -73.7178  610.5767
      |   450.0000  -74.1185  611.1778
      |   450.0000  -74.5174  611.7761
      |   450.0000  -74.9145  612.3717
      |   450.0000  -75.3096  612.9645
      |   450.0000  -75.7029  613.5544
      |   450.0000  -76.0943  614.1414
      |   450.0000  -76.4837  614.7255
      |   450.0000  -76.8711  615.3066
      |   450.0000  -77.2564  615.8846
      |   450.0000  -77.6397  616.4596
      |   450.0000  -78.0209  617.0314
      |   450.0000  -78.4000  617.6000
      |   450.0000  -78.7769  618.1654
      |   450.0000  -79.1516  618.7275
      |   450.0000  -79.5241  619.2862
      |   450.0000  -79.8944  619.8416
      |   450.0000  -80.2623  620.3935
      |   450.0000  -80.6280  620.9419
      |   450.0000  -80.9912  621.4868
      |   450.0000  -81.3521  622.0282
      |   450.0000  -81.7106  622.5659
      |   450.0000  -82.0666  623.0999
      |   450.0000  -82.4201  623.6302
      |   450.0000  -82.7711  624.1567
      |   450.0000  -83.1196  624.6794
      |   450.0000  -83.4655  625.1983
      |   450.0000  -83.8088  625.7132
      |   450.0000  -84.1494  626.2241
      |   450.0000  -84.4873  626.7310
      |   450.0000  -84.8226  627.2339
      |   450.0000  -85.1551  627.7326
      |   450.0000  -85.4848  628.2272
      |   450.0000  -85.8117  628.7176
      |   450.0000  -86.1358  629.2037
      |   450.0000  -86.4570  629.6855
      |   450.0000  -86.7753  630.1629
      |   450.0000  -87.0906  630.6359
      |   450.0000  -87.4030  631.1045
      |   450.0000  -87.7124  631.5686
      |   450.0000  -88.0187  632.0281
      |   450.0000  -88.3220  632.4830
      |   450.0000  -88.6222  632.9333
      |   450.0000  -88.9192  633.3789
      |   450.0000  -89.2131  633.8197
      |   450.0000  -89.5038  634.2557
      |   450.0000  -89.7913  634.6869
      |   450.0000  -90.0755  635.1132
      |   450.0000  -90.3564  635.5346
      |   450.0000  -90.6340  635.9509
      |   450.0000  -90.9082  636.3623
      |   450.0000  -91.1790  636.7685
      |   450.0000  -91.4464  637.1696
      |   450.0000  -91.7103  637.5655
      |   450.0000  -91.9708  637.9562
      |   450.0000  -92.2277  638.3416
      |   450.0000  -92.4811  638.7217
      |   450.0000  -92.7309  639.0964
      |   450.0000  -92.9771  639.4657
      |   450.0000  -93.2196  639.8295
      |   450.0000  -93.4585  640.1877
      |   450.0000  -93.6936  640.5404
      |   450.0000  -93.9250  640.8875
      |   450.0000  -94.1526  641.2289
      |   450.0000  -94.3764  641.5646
      |   450.0000  -94.5963  641.8945
      |   450.0000  -94.8124  642.2186
      |   450.0000  -95.0246  642.5369
      |   450.0000  -95.2328  642.8492
      |   450.0000  -95.4370  643.1556
      |   450.0000  -95.6373  643.4559
      |   450.0000  -95.8335  643.7502
      |   450.0000  -96.0256  644.0384
      |   450.0000  -96.2136  644.3204
      |   450.0000  -96.3975  644.5963
      |   450.0000  -96.5772  644.8658
      |   450.0000  -96.7527  645.1291
      |   450.0000  -96.9240  645.3860
      |   450.0000  -97.0910  645.6366
      |   450.0000  -97.2538  645.8806
      |   450.0000  -97.4121  646.1182
      |   450.0000  -97.5662  646.3493
      |   450.0000  -97.7158  646.5737
      |   450.0000  -97.8610  646.7915
      |   450.0000  -98.0017  647.0026
      |   450.0000  -98.1380  647.2070
      |   450.0000  -98.2697  647.4046
      |   450.0000  -98.3969  647.5953
      |   450.0000  -98.5194  647.7792
      |   450.0000  -98.6374  647.9561
      |   450.0000  -98.7507  648.1260
      |   450.0000  -98.8593  648.2890
      |   450.0000  -98.9632  648.4448
      |   450.0000  -99.0623  648.5935
      |   450.0000  -99.1567  648.7350
      |   450.0000  -99.2462  648.8693
      |   450.0000  -99.3309  648.9964
      |   450.0000  -99.4107  649.1161
      |   450.0000  -99.4856  649.2284
      |   450.0000  -99.5556  649.3333
      |   450.0000  -99.6205  649.4308
      |   450.0000  -99.6805  649.5207
      |   450.0000  -99.7354  649.6031
      |   450.0000  -99.7852  649.6779
      |   450.0000  -99.8300  649.7449
      |   450.0000  -99.8696  649.8043
      |   450.0000  -99.9040  649.8559
      |   450.0000  -99.9332  649.8998
      |   450.0000  -99.9571  649.9357
      |   450.0000  -99.9758  649.9638
      |   450.0000  -99.9892  649.9839
      |   450.0000  -99.9973  649.9960
      |   450.0000 -100.0000  650.0000]
  Sum : Sum  Inputs=+-
  Sum1 : Sum  Inputs=+-
  Sum2 : Sum  Inputs=+-
  Sum3 : Sum  Inputs=-+
  Sum4 : Sum  Inputs=-+
  Sum5 : Sum  Inputs=-+
  Transform : sm_lib/Frames and Transforms/Rigid Transform  TranslationMethod=Cartesian  TranslationStandardOffset=0  TranslationLengthUnit=mm  TranslationStandardAxis=+Z  TranslationCartesianOffset=smiData.RigidTransform(13).translation  TranslationROffset=0  TranslationROffsetUnits=m  TranslationZOffset=0  TranslationZOffsetUnits=m  TranslationThetaOffset=0  TranslationThetaOffsetUnits=deg  RotationMethod=ArbitraryAxis  RotationAngleUnits=rad  RotationStandardAxis=+Z  RotationAngle=smiData.RigidTransform(13).angle  RotationArbitraryAxis=smiData.RigidTransform(13).axis  FollAlignAxisA=+X  BaseAlignAxisA=+Y  FollAlignAxisB=+Y  BaseAlignAxisB=+Z  RotationSequenceAxes=FollowerAxes  RotationSequence=XYX  RotationSequenceAngles=[0 0 0]  RotationSequenceAnglesUnits=deg  RotationMatrix=[1 0 0; 0 1 0; 0 0 1]
  World : sm_lib/Frames and Transforms/World Frame
  base_4_RIGID : Subsystem
  link1_1_RIGID : Subsystem
  link2_1_RIGID : Subsystem
  link3_1_RIGID : Subsystem
  link4_1_RIGID : Subsystem
  link5_test1_1_RIGID : Subsystem
  link5_test2_2_RIGID : Subsystem
  the : Outport
  wires:
  [the2_r] -> Simulink-PS Converter1/1
  Sum2/1 -> Simulink-PS Converter5/1
  [the4_r] -> Simulink-PS Converter3/1
  Constant17/1 -> Simulink-PS Converter5/3
  Constant12/1 -> Sum1/1
  Constant5/1 -> Simulink-PS Converter1/3
  Constant7/1 -> Simulink-PS Converter2/2
  [the6_r] -> Sum2/2
  Constant1/1 -> Simulink-PS Converter/2
  Sum1/1 -> Simulink-PS Converter4/1
  Constant13/1 -> Simulink-PS Converter4/2
  Sum/1 -> Simulink-PS Converter2/1
  Constant15/1 -> Sum2/1
  Constant16/1 -> Simulink-PS Converter5/2
  Constant11/1 -> Simulink-PS Converter3/3
  Constant10/1 -> Simulink-PS Converter3/2
  [the5_r] -> Sum1/2
  [the3_r] -> Sum/2
  Constant18/1 -> Sum/1
  [the1_r] -> Simulink-PS Converter/1
  Constant2/1 -> Simulink-PS Converter/3
  Constant4/1 -> Simulink-PS Converter1/2
  Constant14/1 -> Simulink-PS Converter4/3
  Constant8/1 -> Simulink-PS Converter2/3
  the_r/1 -> Demux/1
  Demux/1 -> [the1_r]
  Demux/2 -> [the2_r]
  Demux/3 -> [the3_r]
  Demux/4 -> [the4_r]
  Demux/5 -> [the5_r]
  Demux/6 -> [the6_r]
  PS-Simulink Converter1/1 -> [the1]
  PS-Simulink Converter2/1 -> [the2]
  PS-Simulink Converter4/1 -> [the4]
  Sum4/1 -> [the5]
  Sum5/1 -> [the6]
  [the1] -> Mux/1
  [the2] -> Mux/2
  [the3] -> Mux/3
  [the4] -> Mux/4
  [the5] -> Mux/5
  [the6] -> Mux/6
  Mux/1 -> the/1
  PS-Simulink Converter3/1 -> Sum3/1
  Constant3/1 -> Sum3/2
  Sum3/1 -> [the3]
  PS-Simulink Converter5/1 -> Sum4/1
  Constant6/1 -> Sum4/2
  PS-Simulink Converter6/1 -> Sum5/1
  Constant9/1 -> Sum5/2
  connections:
  Revolute5/LConn1 -- link5_test1_1_RIGID/RConn1
  Revolute2/LConn1 -- link2_1_RIGID/RConn1
  MechanismConfiguration/RConn1 -- Solver Configuration/RConn1 -- World/RConn1 -- Spline/LConn1 -- Transform/LConn1
  Simulink-PS Converter/RConn1 -- Revolute/LConn2
  Revolute5/RConn1 -- link5_test2_2_RIGID/LConn1
  Revolute/RConn1 -- link1_1_RIGID/LConn1
  Revolute1/LConn1 -- link1_1_RIGID/RConn1
  Revolute3/LConn2 -- Simulink-PS Converter3/RConn1
  Revolute2/RConn1 -- link3_1_RIGID/LConn1
  Revolute1/RConn1 -- link2_1_RIGID/LConn1
  Revolute4/RConn1 -- link5_test1_1_RIGID/LConn1
  Revolute3/LConn1 -- link3_1_RIGID/RConn1
  Revolute4/LConn1 -- link4_1_RIGID/RConn1
  Revolute/LConn1 -- base_4_RIGID/RConn1
  Revolute4/LConn2 -- Simulink-PS Converter4/RConn1
  Revolute3/RConn1 -- link4_1_RIGID/LConn1
  Revolute2/LConn2 -- Simulink-PS Converter2/RConn1
  Revolute1/LConn2 -- Simulink-PS Converter1/RConn1
  Revolute5/LConn2 -- Simulink-PS Converter5/RConn1
  Transform/RConn1 -- base_4_RIGID/LConn1
  Revolute/RConn2 -- PS-Simulink Converter1/LConn1
  Revolute1/RConn2 -- PS-Simulink Converter2/LConn1
  Revolute2/RConn2 -- PS-Simulink Converter3/LConn1
  Revolute3/RConn2 -- PS-Simulink Converter4/LConn1
  Revolute4/RConn2 -- PS-Simulink Converter5/LConn1
  Revolute5/RConn2 -- PS-Simulink Converter6/LConn1
